simulink model "regenerative_damper_make_picture"  (R2017a)
settings: Solver=ode45  StartTime=0.0  StopTime=0.3  MaxStep=1e-5  RelTol=1e-4
libraries: powerlib_meascontrol x4, pe_lib x4, fl_lib x2, elec_lib x1
settings Model: Creator=k1506456  LastModifiedBy=k1506456

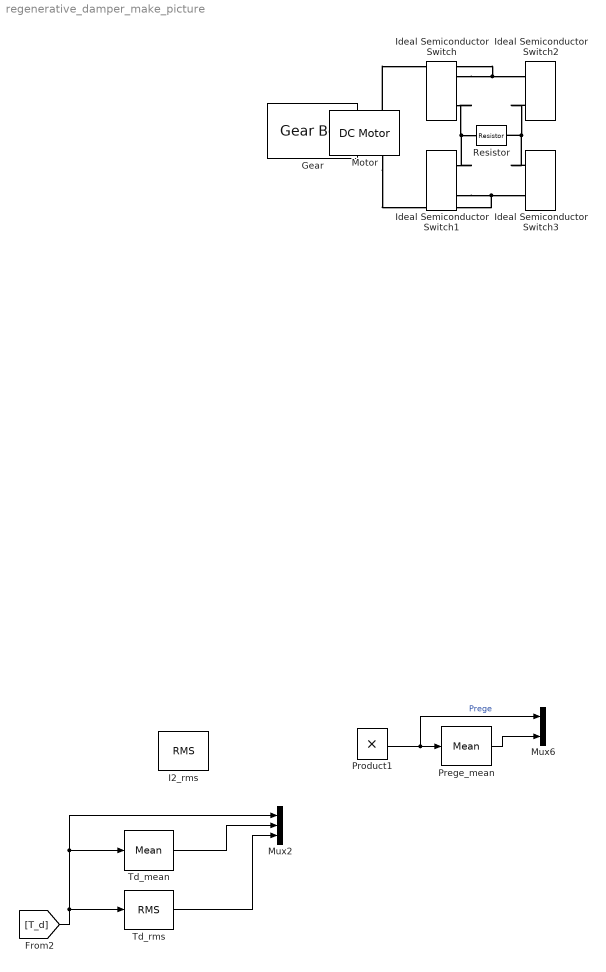
== system regenerative_damper_make_picture ==
  Gear : fl_lib/Mechanical/Mechanisms/Gear Box  ratio=5  t_in_specify=off  t_in_priority=None  t_in=0 N*m  t_in_nominal_specify=off  t_in_nominal_unit=N*m  t_in_nominal_value=1  t_out_specify=off  t_out_priority=None  t_out=0 N*m  t_out_nominal_specify=off  t_out_nominal_unit=N*m  t_out_nominal_value=1  mask(Gear Box){}
      mask Display: image('C:\Users\k1506456\Pictures\2gears.PNG');
  I2_rms : powerlib_meascontrol/Measurements/RMS  TrueRMS=on  Freq=50  RMSInit=0  Ts=0
  Ideal Semiconductor Switch{,1..3} (4 alike) : pe_lib/Semiconductors/Fundamental Components/Ideal Semiconductor Switch  Ron=0.001 Ohm  Goff=1e-6 1/Ohm  Vth=0.5 V  diode_param=1  diode_Vf=0.8 V  diode_Ron=0.001 Ohm  diode_Goff=1e-5 1/Ohm  diode_C=5e-8 F  diode_iRM=-235 A  diode_iF=300 A  diode_idot=-50 A/us  diode_trr_param=1  diode_trr_factor=3  diode_trr=15 us  diode_Qrr=1.5e+3 s*uA
      settings: SourceProductName=Simscape Power Systems  SourceProductBaseCode=PS
  Motor : elec_lib/Actuators & Drivers/Rotational Actuators/DC Motor  parameterization=1  Ra=21.2 Ohm  La=1.37 mH  emf_or_torque=2  Kv=0.00222222 V/rpm  Ki=0.0212 N*m/A  T_stall=2.4e-4 N*m  w_max=1.91e+4 rpm  w_rated=1.5e+4 rpm  P_rated=0.08 W  V_rated=1.5 V  J=4.2 g*cm^2  lam_param=2  lam=0 N*m/(rad/s)  i_noload=8.81 mA  V_i_noload=24 V  speed0=0 rpm  alpha=0.00393 1/K  Tmeas=25 degC  thermal_mass=100 J/K  initial_temperature=25 degC
  Mux2 : Mux  Inputs=3
  Mux6 : Mux  Inputs=2
  Prege_mean : powerlib_meascontrol/Measurements/Mean  Freq=50  Vinit=0  Ts=0
  Product1 : Product
  Resistor : fl_lib/Electrical/Electrical Elements/Resistor  R=21.2 Ohm  i_specify=off  i_priority=None  i=0 A  i_nominal_specify=off  i_nominal_unit=A  i_nominal_value=1  v_specify=off  v_priority=None  v=0 V  v_nominal_specify=off  v_nominal_unit=V  v_nominal_value=1
  Td_mean : powerlib_meascontrol/Measurements/Mean  Freq=50  Vinit=0  Ts=0
  Td_rms : powerlib_meascontrol/Measurements/RMS  TrueRMS=on  Freq=50  RMSInit=0  Ts=0
  wires:
  [T_d] -> Mux2/1, Td_mean/1, Td_rms/1
  Td_mean/1 -> Mux2/2
  Td_rms/1 -> Mux2/3
  Product1/1 -> Prege_mean/1, Mux6/1  "Prege"
  Prege_mean/1 -> Mux6/2
  connections:
  Ideal Semiconductor Switch2/RConn2 -- Ideal Semiconductor Switch3/RConn1 -- Resistor/RConn1
  Ideal Semiconductor Switch1/RConn2 -- Motor/RConn1 -- Ideal Semiconductor Switch3/RConn2
  Ideal Semiconductor Switch/RConn2 -- Ideal Semiconductor Switch1/RConn1 -- Resistor/LConn1
  Ideal Semiconductor Switch/RConn1 -- Motor/LConn1 -- Ideal Semiconductor Switch2/RConn1
